simulink model "modelo_roll_4dof"  (R2025a)
settings: Solver=VariableStepAuto  StartTime=0.0  StopTime=10.0  RelTol=1e-3
undefined symbols (not defined in the file): a, b, C_phi_total, delta_input, Fz_f_static, Fz_r_static, h_rc, Ix, Iz, K_phi_f, K_phi_r, K_phi_total, m, ms, t_f, t_r, vx
settings Model: Creator=Anderson  LastModifiedBy=Anderson

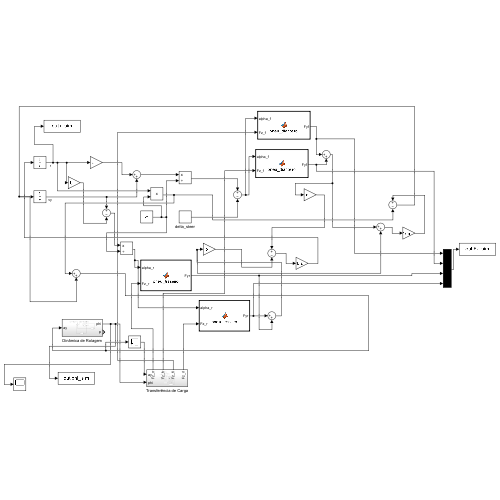
[thumbnail: Simulink's stored preview of the top-level diagram]
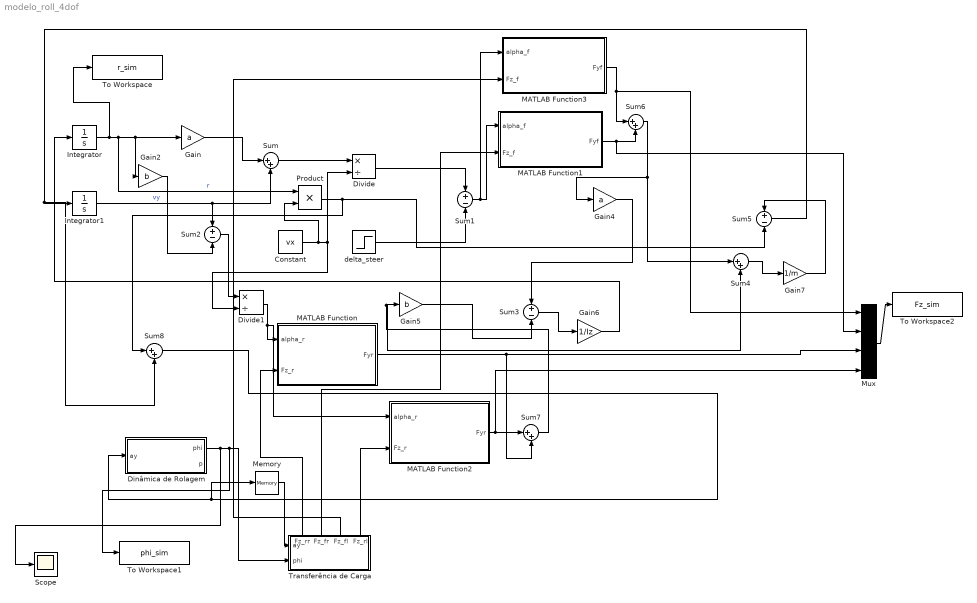
== system modelo_roll_4dof ==
  Constant : Constant  Value=vx
  Dinâmica de Rolagem : Subsystem
  Divide : Product  Inputs=*/
  Divide1 : Product  Inputs=*/
  Gain : Gain  Gain=a
  Gain2 : Gain  Gain=b
  Gain4 : Gain  Gain=a
  Gain5 : Gain  Gain=b
  Gain6 : Gain  Gain=1/Iz
  Gain7 : Gain  Gain=1/m
  Integrator : Integrator
  Integrator1 : Integrator
  MATLAB Function : MATLAB Function  TreatAsAtomicUnit=on
  MATLAB Function1 : MATLAB Function  TreatAsAtomicUnit=on
  MATLAB Function2 : MATLAB Function  TreatAsAtomicUnit=on
  MATLAB Function3 : MATLAB Function  TreatAsAtomicUnit=on
  Memory : Memory
  Mux : Mux
  Product : Product
  Scope : Scope
      settings: ActiveDisplayYMinimum=-0.015845896943885822  ActiveDisplayYMaximum=0.10203921668817159
  Sum{,4,6..8} (5 alike) : Sum  Inputs=|++
  Sum{1..3,5} (4 alike) : Sum  Inputs=+-
  To Workspace : ToWorkspace  VariableName=r_sim  SaveFormat=Timeseries  SampleTime=-1
  To Workspace1 : ToWorkspace  VariableName=phi_sim  SaveFormat=Timeseries  SampleTime=-1
  To Workspace2 : ToWorkspace  VariableName=Fz_sim  SaveFormat=Timeseries  SampleTime=-1
  Transferência de Carga : Subsystem
      settings: PortSchema="{\"entries\":[{\"content\":{\"sides\":[{\"content\":{\"connectorIds\":[\"In1\",\"In2\"]},\"type\":\"ConnectorPlacement.EquallySpacedRectSide\",\"uuid\":\"e925ad76-6aec-44f5-ab0f-a760dba7f5fe\"},{\"content\":{\"side\":\"RIGHT\"},\"type\":\"ConnectorPlacement.EquallySpacedRectSide\",\"uuid\":\"3825e0e8-9ec4-4f20-b740-9c23807b7287\"},{\"content\":{\"connectorIds\":[\"Out1\",\"Out2\",\"Out3\",\"Out4\"],\"side\":\"TOP\"},\"type\":\"ConnectorPlacement.EquallySpacedRectSide\",\"uuid\":\"5d8f76d2-4569-4618-8574-d5788c526c3e\"}]},\"type\":\"ConnectorPlacement.EquallySpacedConnector\",\"uuid\":\"9a321bb4-cdbe-47ff-9619-cf02739e8cce\"}],\"packageUris\":[\"http://schema.mathworks.com/mf0/Connector/R2020b\"],\"version\":\"1.0\"}"
  delta_steer : Step  After=delta_input  SampleTime=0
  wires:
  Integrator/1 -> To Workspace/1, Product/1, Gain2/1, Gain/1  "r"
  Integrator1/1 -> Sum2/1, Sum/2  "vy"
  Gain/1 -> Sum/1
  Sum/1 -> Divide/1
  Constant/1 -> Product/2, Divide1/2, Divide/2
  Divide/1 -> Sum1/1
  delta_steer/1 -> Sum1/2
  Sum1/1 -> MATLAB Function3/1(alpha_f), MATLAB Function1/1(alpha_f)
  Gain2/1 -> Sum2/2
  Gain4/1 -> Sum3/1
  Gain5/1 -> Sum3/2
  Sum3/1 -> Gain6/1
  Gain6/1 -> Integrator/1
  Sum4/1 -> Gain7/1
  Gain7/1 -> Sum5/1
  Product/1 -> Sum8/1, Sum5/2
  Sum5/1 -> Sum8/2, Integrator1/1
  Sum2/1 -> Divide1/1
  Divide1/1 -> MATLAB Function2/1(alpha_r), MATLAB Function/1(alpha_r)
  MATLAB Function1/1(Fyf) -> Mux/2, Sum6/2
  Sum6/1 -> Sum4/1, Gain4/1
  MATLAB Function2/1(Fyr) -> Mux/4, Sum7/1
  MATLAB Function/1(Fyr) -> Mux/3, Sum7/2
  Sum7/1 -> Sum4/2, Gain5/1
  Sum8/1 -> Memory/1, Dinâmica de Rolagem/1(ay)
  Dinâmica de Rolagem/1(phi) -> Scope/1, To Workspace1/1, Transferência de Carga/2(phi)
  Transferência de Carga/4(Fz_rl) -> MATLAB Function2/2(Fz_r)
  Transferência de Carga/1(Fz_rr) -> MATLAB Function/2(Fz_r)
  Transferência de Carga/2(Fz_fr) -> MATLAB Function1/2(Fz_f)
  Transferência de Carga/3(Fz_fl) -> MATLAB Function3/2(Fz_f)
  MATLAB Function3/1(Fyf) -> Mux/1, Sum6/1
  Mux/1 -> To Workspace2/1
  Memory/1 -> Transferência de Carga/1(ay)

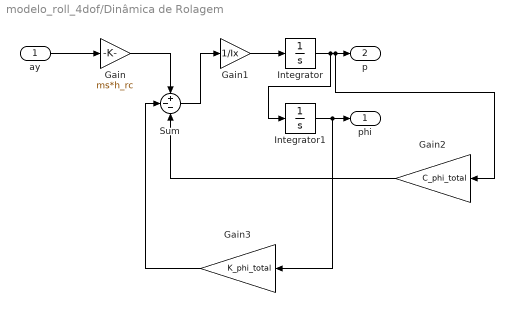
== system modelo_roll_4dof/Dinâmica de Rolagem ==
  ay : Inport
  Gain : Gain  Gain=ms*h_rc
  Gain1 : Gain  Gain=1/Ix
  Gain2 : Gain  Gain=C_phi_total
  Gain3 : Gain  Gain=K_phi_total
  Integrator : Integrator
  Integrator1 : Integrator
  Sum : Sum  Inputs=+--
  phi : Outport
  p : Outport  Port=2
  wires:
  ay/1 -> Gain/1
  Gain/1 -> Sum/1
  Sum/1 -> Gain1/1
  Gain1/1 -> Integrator/1
  Integrator/1 -> Integrator1/1, Gain2/1, p/1
  Integrator1/1 -> Gain3/1, phi/1
  Gain3/1 -> Sum/2
  Gain2/1 -> Sum/3

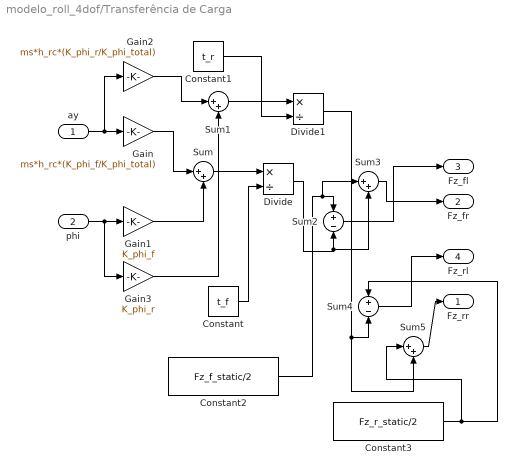
== system modelo_roll_4dof/Transferência de Carga ==
  ay : Inport
  phi : Inport  Port=2
  Constant : Constant  Value=t_f
  Constant1 : Constant  Value=t_r
  Constant2 : Constant  Value=Fz_f_static/2
  Constant3 : Constant  Value=Fz_r_static/2
  Divide : Product  Inputs=*/
  Divide1 : Product  Inputs=*/
  Gain : Gain  Gain=ms*h_rc*(K_phi_f/K_phi_total)
  Gain1 : Gain  Gain=K_phi_f
  Gain2 : Gain  Gain=ms*h_rc*(K_phi_r/K_phi_total)
  Gain3 : Gain  Gain=K_phi_r
  Sum{,1,3,5} (4 alike) : Sum  Inputs=|++
  Sum2 : Sum  Inputs=+-
  Sum4 : Sum  Inputs=+-
  Fz_rr : Outport
  Fz_fr : Outport  Port=2
  Fz_fl : Outport  Port=3
  Fz_rl : Outport  Port=4
  wires:
  ay/1 -> Gain2/1, Gain/1
  phi/1 -> Gain3/1, Gain1/1
  Gain/1 -> Sum/1
  Gain1/1 -> Sum/2
  Sum/1 -> Divide/1
  Constant/1 -> Divide/2
  Gain2/1 -> Sum1/1
  Gain3/1 -> Sum1/2
  Constant1/1 -> Divide1/2
  Sum1/1 -> Divide1/1
  Constant2/1 -> Sum3/1, Sum2/1
  Sum2/1 -> Fz_fl/1
  Sum3/1 -> Fz_fr/1
  Divide/1 -> Sum3/2, Sum2/2
  Constant3/1 -> Sum5/1, Sum4/1
  Divide1/1 -> Sum5/2, Sum4/2
  Sum4/1 -> Fz_rl/1
  Sum5/1 -> Fz_rr/1

== matlab function modelo_roll_4dof/MATLAB Function ==
  data: alpha_r input; Fyr output; Fz_r input
function Fyr = pneu_traseiro(alpha_r, Fz_r)
% CÓDIGO CORRIGIDO COM INICIALIZAÇÃO

Fyr = 0.0; % <-- ADICIONE ESTA LINHA: Pré-inicializa a variável de saída

% Coeficientes de Pacejka definidos diretamente aqui dentro
B = 10;
C = 1.9;
D_mult = 1.0;
E = 0.97;

% O pico da aderência (D) depende da carga vertical (Fz)
D = D_mult * Fz_r;

% Magic Formula de Pacejka (usando radianos)
phi = (1 - E) * alpha_r + (E / B) * atan(B * alpha_r);
Fyr_mag = D * sin(C * atan(B * phi));

% A força lateral é oposta ao ângulo de deriva
Fyr = -Fyr_mag;

end

== matlab function modelo_roll_4dof/MATLAB Function2 ==
  data: alpha_r input; Fyr output; Fz_r input
function Fyr = pneu_traseiro(alpha_r, Fz_r)
% CÓDIGO CORRIGIDO COM INICIALIZAÇÃO

Fyr = 0.0; % <-- ADICIONE ESTA LINHA: Pré-inicializa a variável de saída

% Coeficientes de Pacejka definidos diretamente aqui dentro
B = 10;
C = 1.9;
D_mult = 1.0;
E = 0.97;

% O pico da aderência (D) depende da carga vertical (Fz)
D = D_mult * Fz_r;

% Magic Formula de Pacejka (usando radianos)
phi = (1 - E) * alpha_r + (E / B) * atan(B * alpha_r);
Fyr_mag = D * sin(C * atan(B * phi));

% A força lateral é oposta ao ângulo de deriva
Fyr = -Fyr_mag;

end

== matlab function modelo_roll_4dof/MATLAB Function3 ==
  data: alpha_f input; Fyf output; Fz_f input
function Fyf = pneu_dianteiro(alpha_f, Fz_f)
% CÓDIGO CORRIGIDO COM INICIALIZAÇÃO

Fyf = 0.0; % <-- ADICIONE ESTA LINHA: Pré-inicializa a variável de saída

% Coeficientes de Pacejka definidos diretamente aqui dentro
B = 10;
C = 1.9;
D_mult = 1.0;
E = 0.97;

% O pico da aderência (D) depende da carga vertical (Fz)
D = D_mult * Fz_f;

% Magic Formula de Pacejka (usando radianos)
phi = (1 - E) * alpha_f + (E / B) * atan(B * alpha_f);
Fyf_mag = D * sin(C * atan(B * phi));

% A força lateral é oposta ao ângulo de deriva
Fyf = -Fyf_mag;

end

== matlab function modelo_roll_4dof/MATLAB Function1 ==
  data: alpha_f input; Fyf output; Fz_f input
function Fyf = pneu_dianteiro(alpha_f, Fz_f)
% CÓDIGO CORRIGIDO COM INICIALIZAÇÃO

Fyf = 0.0; % <-- ADICIONE ESTA LINHA: Pré-inicializa a variável de saída

% Coeficientes de Pacejka definidos diretamente aqui dentro
B = 10;
C = 1.9;
D_mult = 1.0;
E = 0.97;

% O pico da aderência (D) depende da carga vertical (Fz)
D = D_mult * Fz_f;

% Magic Formula de Pacejka (usando radianos)
phi = (1 - E) * alpha_f + (E / B) * atan(B * alpha_f);
Fyf_mag = D * sin(C * atan(B * phi));

% A força lateral é oposta ao ângulo de deriva
Fyf = -Fyf_mag;

end
